simulink model "part3model"  (R2019b)
settings: Solver=VariableStepAuto  StartTime=0.0  StopTime=4  RelTol=1e-3
values from neighbouring files (symbols this model uses):
  encGain = (2*pi)/4096    (= 0.00153398078789)    [DC_Motor_Analysis.m]    (also in Part2.m; Part3.m; lqrPoles.mat; robust.mat)
  K_rt = K(1:2).'    [Part3.m]
  ka = K(end)    [Part3.m]    (also in Part4.m; lqrPoles.mat = 316.227766017)
settings Model: Creator=justinf  LastModifiedBy=justinf
settings DebuggingCC: AlgebraicLoopMsg=none

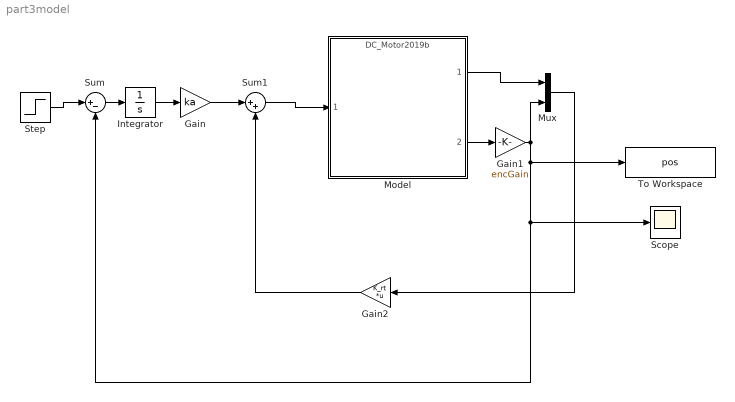
== system part3model ==
  Gain : Gain  Gain=ka
  Gain1 : Gain  Gain=encGain
  Gain2 : Gain  Gain=K_rt  Multiplication=Matrix(K*u) (u vector)
  Integrator : Integrator
  Model : ModelReference  ModelNameDialog=DC_Motor2019b.slxp  ModelReferenceVersion=1.20  CopyOfModelProtected=on
  Mux : Mux  Inputs=2
  Scope : Scope
  Step : Step  Time=0  SampleTime=0
  Sum : Sum  Inputs=|+-
  Sum1 : Sum  Inputs=|++
  To Workspace : ToWorkspace  VariableName=pos  SampleTime=-1
  wires:
  Sum1/1 -> Model/1
  Gain/1 -> Sum1/1
  Integrator/1 -> Gain/1
  Sum/1 -> Integrator/1
  Step/1 -> Sum/1
  Model/2 -> Gain1/1
  Gain2/1 -> Sum1/2
  Model/1 -> Mux/1
  Gain1/1 -> Mux/2, To Workspace/1, Scope/1, Sum/2
  Mux/1 -> Gain2/1
